simulink model "Task_4"  (R2021b)
settings: Solver=FixedStepDiscrete  StartTime=0.0  StopTime=100.0  FixedStep=0.01  RelTol=1e-3
model workspace (MAT data in the model file):
  Kd = 2
  Ki = 300
  Kp = 600
  Ts = 0.01
settings Model: Creator=mluser  LastModifiedBy=mluser
settings OptimizationCC: DefaultParameterBehavior=Inlined  EnhancedBackFolding=on  PassReuseOutputArgsAs=Individual arguments  ZeroExternalMemoryAtStartup=off  ZeroInternalMemoryAtStartup=off  OptimizeBlockOrder=speed  DifferentSizesBufferReuse=on  OptimizationCustomize=off  EfficientTunableParamExpr=on
settings DebuggingCC: ParameterTunabilityLossMsg=error
settings SFSimCC: MATLABDynamicMemAlloc=off
settings RTWCC: Description=Embedded Coder  SystemTargetFile=ert.tlc  GenCodeOnly=on  TemplateMakefile=ert_default_tmf  GenerateReport=on  LaunchReport=on
settings CodeAppCC: ForceParamTrailComments=on  IgnoreCustomStorageClasses=off  OperatorAnnotations=on  SimulinkDataObjDesc=on  SFDataObjDesc=on  InsertBlockDesc=on
settings ERTTargetCC: TargetLangStandard=C99 (ISO)  GenerateSampleERTMain=on  InlinedParameterPlacement=NonHierarchical  ERTCustomFileTemplate=example_file_process.tlc

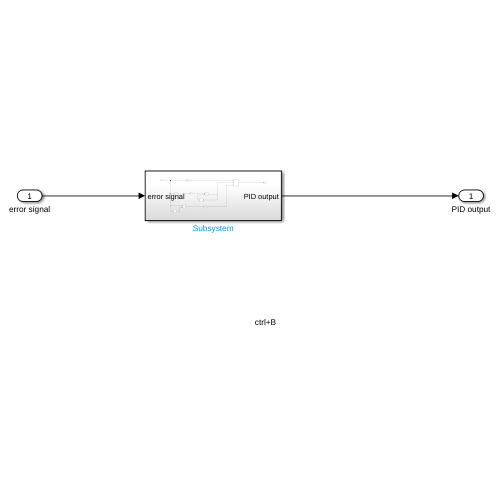
[thumbnail: Simulink's stored preview of the top-level diagram]
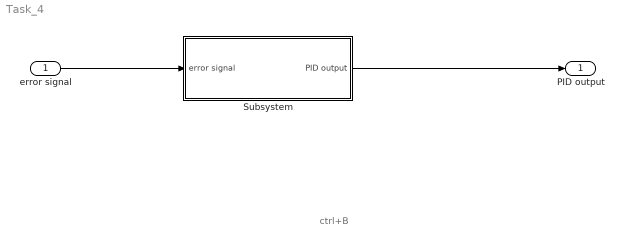
== system Task_4 ==
  note: ctrl+B
  error signal : Inport
  Subsystem : Subsystem
  PID output : Outport
  wires:
  error signal/1 -> Subsystem/1(error signal)
  Subsystem/1(PID output) -> PID output/1

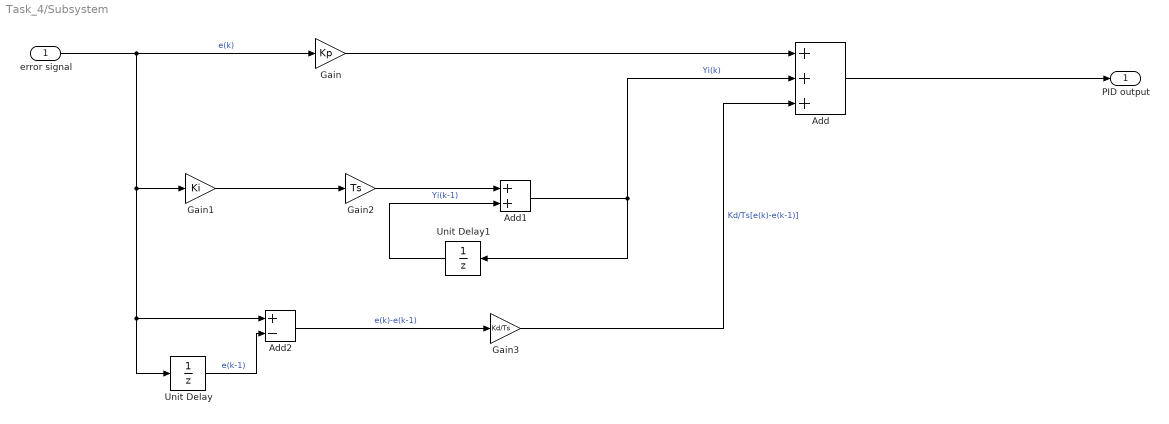
== system Task_4/Subsystem ==
  error signal : Inport
  Add : Sum  Inputs=+++
  Add1 : Sum
  Add2 : Sum  Inputs=+-
  Gain : Gain  Gain=Kp
  Gain1 : Gain  Gain=Ki
  Gain2 : Gain  Gain=Ts
  Gain3 : Gain  Gain=Kd/Ts
  Unit Delay : UnitDelay  SampleTime=-1  HasFrameUpgradeWarning=on
  Unit Delay1 : UnitDelay  SampleTime=-1  HasFrameUpgradeWarning=on
  PID output : Outport
  wires:
  Unit Delay1/1 -> Add1/2  "Yi(k-1)"
  Gain3/1 -> Add/3  "Kd/Ts[e(k)-e(k-1)]"
  Gain1/1 -> Gain2/1
  Unit Delay/1 -> Add2/2  "e(k-1)"
  Gain/1 -> Add/1
  error signal/1 -> Add2/1, Unit Delay/1, Gain1/1, Gain/1  "e(k)"
  Add/1 -> PID output/1
  Add2/1 -> Gain3/1  "e(k)-e(k-1)"
  Add1/1 -> Add/2, Unit Delay1/1  "Yi(k)"
  Gain2/1 -> Add1/1
